simulink model "RTW_3_cluster_follow_system"  (R2016a)
settings: Solver=ode5  StartTime=0.0  StopTime=10  FixedStep=0.001  RelTol=1e-3
values from neighbouring files (symbols this model uses):
  LK1 = [-1 0;0 -1]    [RTW_2_round_system_m.m]    (also in RTW_3_cluster_follow_system_m.m = -LK1; car_m.m = [-1 0;0 -1]')
  M = [1 1;1 -1]    [RTW_3_cluster_follow_system_m.m]
  x0 = [0 0]'    [RTW_2_round_system_m.m]    (also in RTW_3_cluster_follow_system_m.m = x0'; car_m.m = [1 3]')
  x02 = [x0(1) x0(3) x0(5) x0(7) x0(2) x0(4) x0(6) x0(8)]    [RTW_3_cluster_follow_system_m.m]
  xd = [10 10]    [RTW_2_round_system_m.m]    (also in RTW_3_cluster_follow_system_m.m = [0 0 0 0 0 0 0 0]; car_m.m)
libraries: simulink x1
settings Model: Creator=108  LastModifiedBy=richa

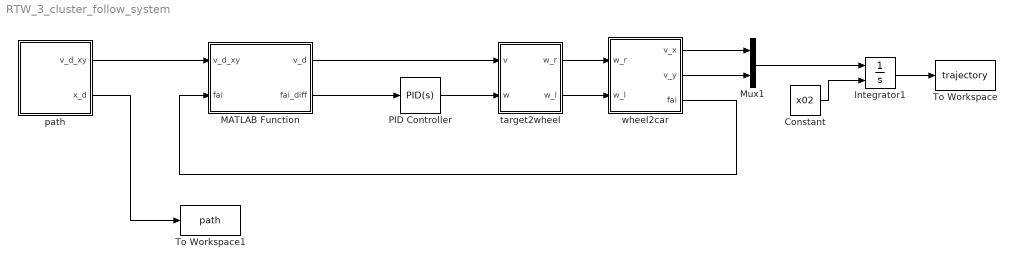
== system RTW_3_cluster_follow_system ==
  Constant : Constant  Value=x02
  Integrator1 : Integrator  InitialConditionSource=external
  MATLAB Function : MATLAB Function  TreatAsAtomicUnit=on
  Mux1 : Mux  Inputs=2
  PID Controller : simulink/Continuous/PID Controller  Controller=PID  TimeDomain=Continuous-time  SampleTime=-1  IntegratorMethod=Forward Euler  FilterMethod=Forward Euler  Form=Parallel  UseFilter=on  ControllerParametersSource=internal  P=200  I=10  D=0  N=100  InitialConditionSource=internal  InitialConditionForIntegrator=0  InitialConditionForFilter=0  ExternalReset=none  LimitOutput=off  UpperSaturationLimit=inf  LowerSaturationLimit=-inf  LinearizeAsGain=on  AntiWindupMode=none  Kb=1  TrackingMode=off  Kt=1  PParamMin=[]  PParamMax=[]  IParamMin=[]  IParamMax=[]  DParamMin=[]  DParamMax=[]  NParamMin=[]  NParamMax=[]  KbParamMin=[]  KbParamMax=[]  KtParamMin=[]  KtParamMax=[]  POutMin=[]  POutMax=[]  IOutMin=[]  IOutMax=[]  DOutMin=[]  DOutMax=[]  NOutMin=[]  NOutMax=[]  KbOutMin=[]  KbOutMax=[]  KtOutMin=[]  KtOutMax=[]  IntegratorOutMin=[]  IntegratorOutMax=[]  FilterOutMin=[]  FilterOutMax=[]  SumOutMin=[]  SumOutMax=[]  SumI1OutMin=[]  SumI1OutMax=[]  SumI2OutMin=[]  SumI2OutMax=[]  SumI3OutMin=[]  SumI3OutMax=[]  SumDOutMin=[]  SumDOutMax=[]  SaturationOutMin=[]  SaturationOutMax=[]  IntegratorContinuousStateAttributes=''  IntegratorStateMustResolveToSignalObject=off  IntegratorRTWStateStorageClass=Auto  FilterContinuousStateAttributes=''  FilterStateMustResolveToSignalObject=off  FilterRTWStateStorageClass=Auto  DifferentiatorICPrevScaledInput=0  DifferentiatorOutMin=[]  DifferentiatorOutMax=[]
  To Workspace : ToWorkspace  VariableName=trajectory  SampleTime=-1
  To Workspace1 : ToWorkspace  VariableName=path  SampleTime=-1
  path : Subsystem
  target2wheel : Subsystem
  wheel2car : Subsystem
  wires:
  target2wheel/1(w_r) -> wheel2car/1(w_r)
  target2wheel/2(w_l) -> wheel2car/2(w_l)
  MATLAB Function/2(fai_diff) -> PID Controller/1
  PID Controller/1 -> target2wheel/2(w)
  wheel2car/3(fai) -> MATLAB Function/2(fai)
  MATLAB Function/1(v_d) -> target2wheel/1(v)
  path/2(x_d) -> To Workspace1/1
  path/1(v_d_xy) -> MATLAB Function/1(v_d_xy)
  Mux1/1 -> Integrator1/1
  Constant/1 -> Integrator1/2
  Integrator1/1 -> To Workspace/1
  wheel2car/1(v_x) -> Mux1/1
  wheel2car/2(v_y) -> Mux1/2

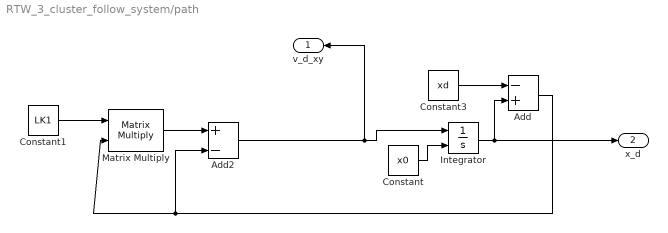
== system RTW_3_cluster_follow_system/path ==
  Add : Sum  Inputs=-+
  Add2 : Sum  Inputs=+-
  Constant : Constant  Value=x0
  Constant1 : Constant  Value=LK1  VectorParams1D=off
  Constant3 : Constant  Value=xd
  Integrator : Integrator  InitialConditionSource=external
  Matrix Multiply : Product  Multiplication=Matrix(*)
  v_d_xy : Outport
  x_d : Outport  Port=2
  wires:
  Matrix Multiply/1 -> Add2/1
  Integrator/1 -> x_d/1, Add/2
  Constant/1 -> Integrator/2
  Constant1/1 -> Matrix Multiply/1
  Add/1 -> Add2/2, Matrix Multiply/2
  Add2/1 -> Integrator/1, v_d_xy/1
  Constant3/1 -> Add/1

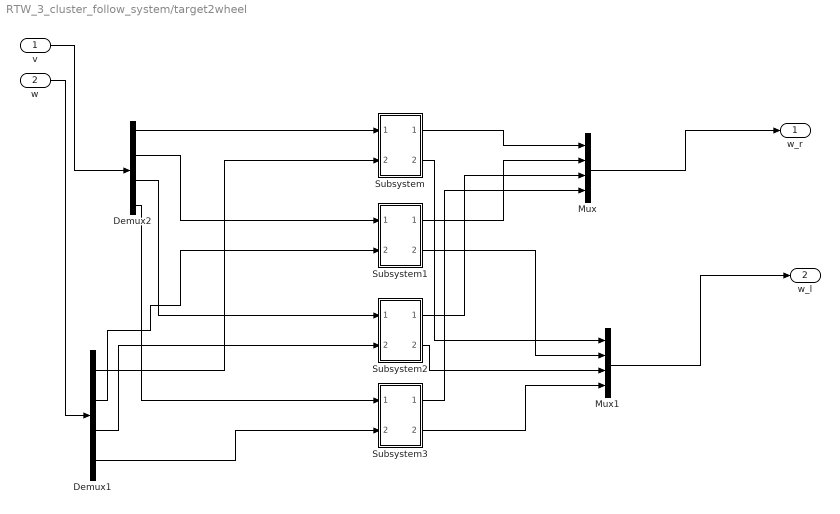
== system RTW_3_cluster_follow_system/target2wheel ==
  v : Inport
  w : Inport  Port=2
  Demux1 : Demux
  Demux2 : Demux
  Mux : Mux
  Mux1 : Mux
  Subsystem : Subsystem
  Subsystem1 : Subsystem
  Subsystem2 : Subsystem
  Subsystem3 : Subsystem
  w_r : Outport
  w_l : Outport  Port=2
  wires:
  v/1 -> Demux2/1
  w/1 -> Demux1/1
  Demux2/2 -> Subsystem1/1(In1)
  Demux2/3 -> Subsystem2/1(In1)
  Demux2/4 -> Subsystem3/1(In1)
  Demux1/2 -> Subsystem1/2(In2)
  Demux1/3 -> Subsystem2/2(In2)
  Demux1/4 -> Subsystem3/2(In2)
  Demux2/1 -> Subsystem/1(In1)
  Demux1/1 -> Subsystem/2(In2)
  Subsystem/1(Out1) -> Mux/1
  Subsystem1/1(Out1) -> Mux/2
  Subsystem2/1(Out1) -> Mux/3
  Subsystem3/1(Out1) -> Mux/4
  Subsystem/2(Out2) -> Mux1/1
  Subsystem1/2(Out2) -> Mux1/2
  Subsystem2/2(Out2) -> Mux1/3
  Subsystem3/2(Out2) -> Mux1/4
  Mux/1 -> w_r/1
  Mux1/1 -> w_l/1

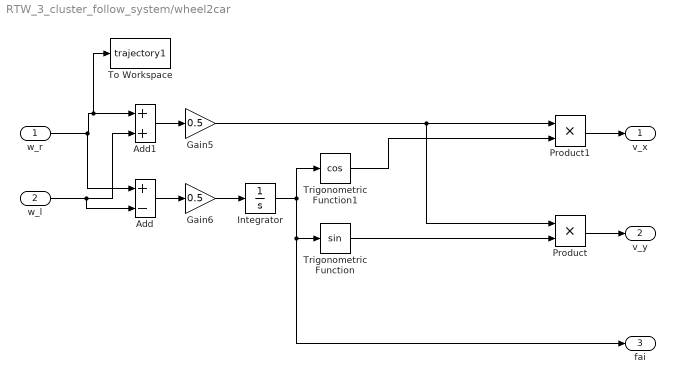
== system RTW_3_cluster_follow_system/wheel2car ==
  w_r : Inport
  w_l : Inport  Port=2
  Add : Sum  Inputs=+-
  Add1 : Sum
  Gain5 : Gain  Gain=0.5
  Gain6 : Gain  Gain=0.5
  Integrator : Integrator
  Product : Product
  Product1 : Product
  To Workspace : ToWorkspace  VariableName=trajectory1  SampleTime=-1
  Trigonometric Function : Trigonometry
  Trigonometric Function1 : Trigonometry  Operator=cos
  v_x : Outport
  v_y : Outport  Port=2
  fai : Outport  Port=3
  wires:
  Gain5/1 -> Product1/1, Product/1
  Gain6/1 -> Integrator/1
  Integrator/1 -> Trigonometric Function1/1, fai/1, Trigonometric Function/1
  Trigonometric Function/1 -> Product/2
  Trigonometric Function1/1 -> Product1/2
  w_r/1 -> Add/1, To Workspace/1, Add1/1
  w_l/1 -> Add/2, Add1/2
  Add1/1 -> Gain5/1
  Add/1 -> Gain6/1
  Product1/1 -> v_x/1
  Product/1 -> v_y/1

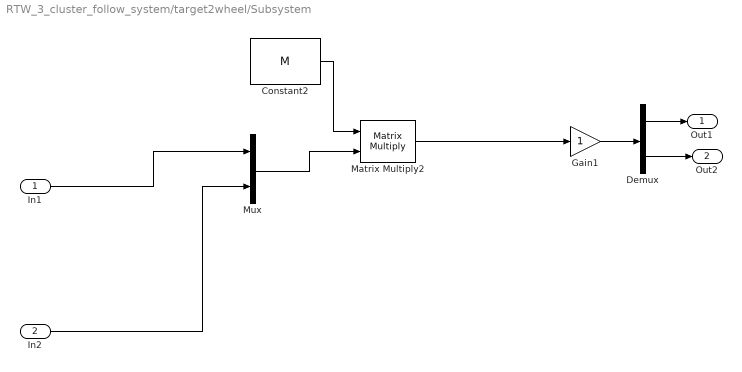
== system RTW_3_cluster_follow_system/target2wheel/Subsystem ==
  In1 : Inport
  In2 : Inport  Port=2
  Constant2 : Constant  Value=M
  Demux : Demux  Outputs=2
  Gain1 : Gain
  Matrix Multiply2 : Product  Multiplication=Matrix(*)
  Mux : Mux  Inputs=2
  Out1 : Outport
  Out2 : Outport  Port=2
  wires:
  Demux/1 -> Out1/1
  In2/1 -> Mux/2
  Mux/1 -> Matrix Multiply2/2
  Gain1/1 -> Demux/1
  In1/1 -> Mux/1
  Matrix Multiply2/1 -> Gain1/1
  Constant2/1 -> Matrix Multiply2/1
  Demux/2 -> Out2/1

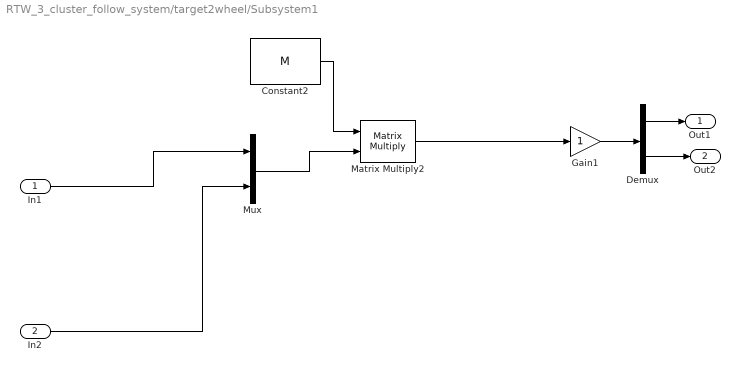
== system RTW_3_cluster_follow_system/target2wheel/Subsystem1 ==
  In1 : Inport
  In2 : Inport  Port=2
  Constant2 : Constant  Value=M
  Demux : Demux  Outputs=2
  Gain1 : Gain
  Matrix Multiply2 : Product  Multiplication=Matrix(*)
  Mux : Mux  Inputs=2
  Out1 : Outport
  Out2 : Outport  Port=2
  wires:
  Demux/2 -> Out2/1
  Constant2/1 -> Matrix Multiply2/1
  Matrix Multiply2/1 -> Gain1/1
  In1/1 -> Mux/1
  Gain1/1 -> Demux/1
  Mux/1 -> Matrix Multiply2/2
  In2/1 -> Mux/2
  Demux/1 -> Out1/1

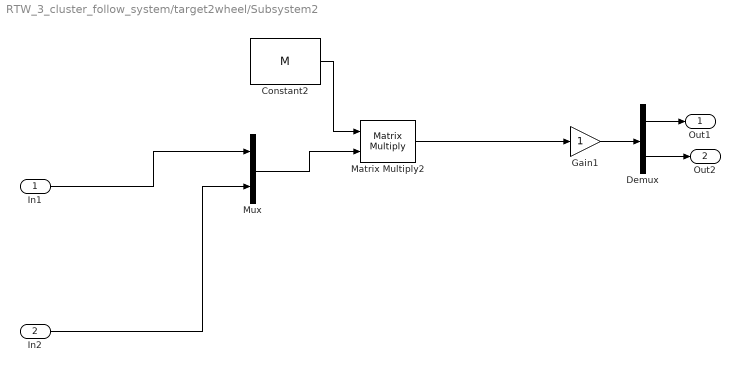
== system RTW_3_cluster_follow_system/target2wheel/Subsystem2 ==
  In1 : Inport
  In2 : Inport  Port=2
  Constant2 : Constant  Value=M
  Demux : Demux  Outputs=2
  Gain1 : Gain
  Matrix Multiply2 : Product  Multiplication=Matrix(*)
  Mux : Mux  Inputs=2
  Out1 : Outport
  Out2 : Outport  Port=2
  wires:
  Demux/1 -> Out1/1
  In2/1 -> Mux/2
  Mux/1 -> Matrix Multiply2/2
  Gain1/1 -> Demux/1
  In1/1 -> Mux/1
  Matrix Multiply2/1 -> Gain1/1
  Constant2/1 -> Matrix Multiply2/1
  Demux/2 -> Out2/1

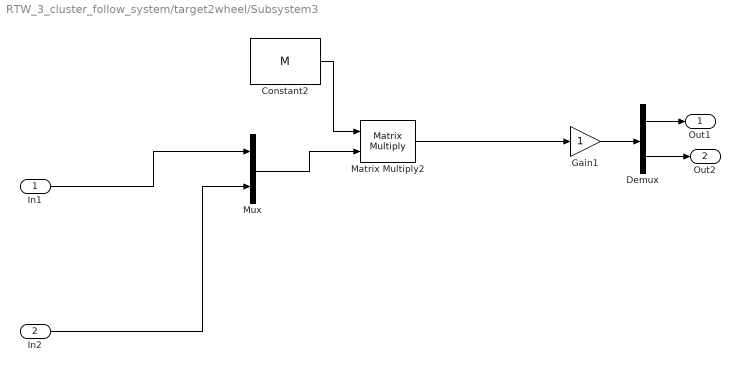
== system RTW_3_cluster_follow_system/target2wheel/Subsystem3 ==
  In1 : Inport
  In2 : Inport  Port=2
  Constant2 : Constant  Value=M
  Demux : Demux  Outputs=2
  Gain1 : Gain
  Matrix Multiply2 : Product  Multiplication=Matrix(*)
  Mux : Mux  Inputs=2
  Out1 : Outport
  Out2 : Outport  Port=2
  wires:
  Demux/2 -> Out2/1
  Constant2/1 -> Matrix Multiply2/1
  Matrix Multiply2/1 -> Gain1/1
  In1/1 -> Mux/1
  Gain1/1 -> Demux/1
  Mux/1 -> Matrix Multiply2/2
  In2/1 -> Mux/2
  Demux/1 -> Out1/1

== matlab function RTW_3_cluster_follow_system/MATLAB Function ==
  data: v_d_xy input; v_d output; fai_diff output; fai input
function [v_d,fai_diff]  = fcn(v_d_xy,fai)
%#codegen

%v_d=[0];
%fai_diff=[0];
v_d=[0 0 0 0];
fai_diff=[0 0 0 0];
fai_d=[0 0 0 0];
j=1;

for i=1:2:7
    v_d(j) = sqrt(v_d_xy(i).^2+ v_d_xy(i+1).^2);
    fai_d(j) = atan2(v_d_xy(i+1),v_d_xy(i));
    fai_diff(j)= fai_d(j)-fai(j);
    if fai_diff(j)>pi
        fai_diff(j)=fai_diff(j)-2*pi*round(fai_diff(j)/(2*pi));
    elseif fai_diff(j)<-pi
        fai_diff(j)=fai_diff(j)+2*pi*round(fai_diff(j)/(-2*pi));      
    end
   
   j=j+1;
end

end
